simulink model "fuzzyLCSv1"  (R2021b)
settings: Solver=VariableStepAuto  StartTime=0.0  StopTime=10  RelTol=1e-3
undefined symbols (not defined in the file or in its folder): NewD, NewI, NewP
libraries: robotlib x3
settings Model: SimulationMode=accelerator  Creator=lucas  LastModifiedBy=lucas

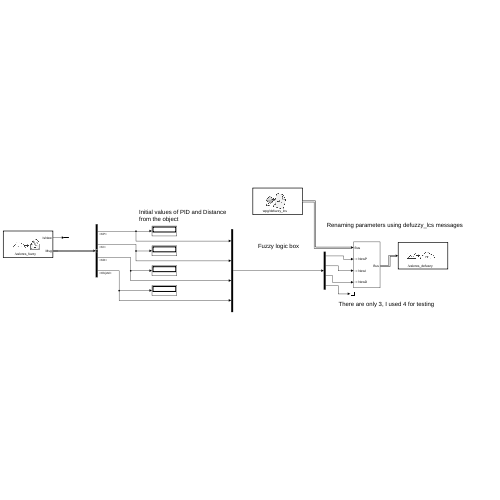
[thumbnail: Simulink's stored preview of the top-level diagram]
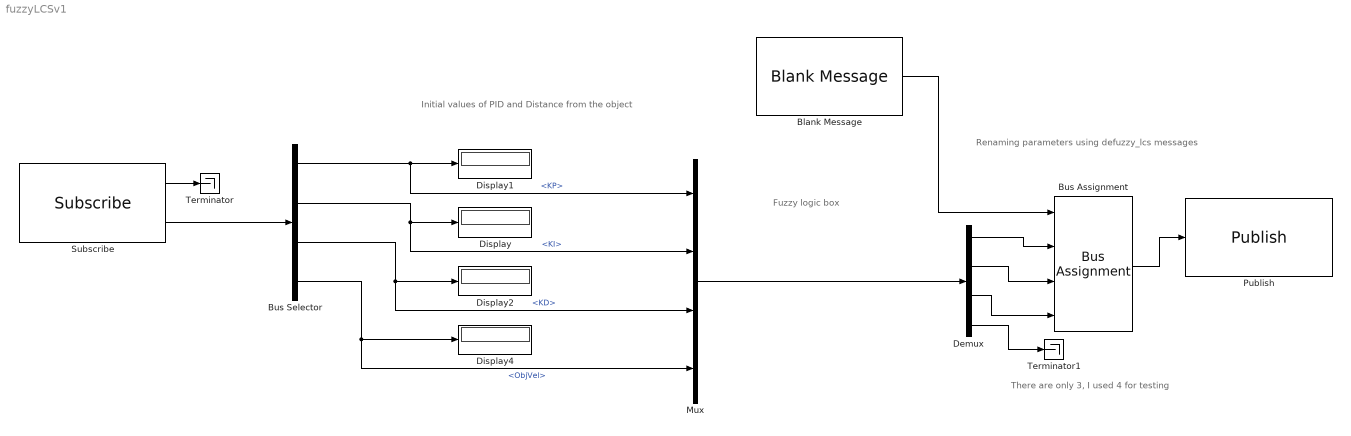
== system fuzzyLCSv1 ==
  note: Renaming parameters using defuzzy_lcs messages
  note: Initial values of PID and Distance
      | from the object
  note: Fuzzy logic box
  note: There are only 3, I used 4 for testing
  Blank Message : robotlib/Blank Message  messageClass=Message  entityType=wpg/defuzzy_lcs  messageType=wpg/defuzzy_lcs  SampleTime=inf  legacyBusStruct=off
  Bus Assignment : BusAssignment  AssignedSignals=NewP,NewI,NewD
  Bus Selector : BusSelector  OutputSignals=KP,KI,KD,ObjVel
  Demux : Demux
  Display{,1..2,4} (4 alike) : Display
      settings: Decimation=2
  Mux : Mux
  Publish : robotlib/Publish  topicSource=Specify your own  topic=/valores_defuzzy  messageType=wpg/defuzzy_lcs  legacyBusStruct=off  messageQueueLength=1
  Subscribe : robotlib/Subscribe  topicSource=Specify your own  topic=/valores_fuzzy  messageType=wpg/fuzzy_lcs  SampleTime=-1  legacyBusStruct=off  messageQueueLength=1
  Terminator : Terminator
  Terminator1 : Terminator
  wires:
  Subscribe/2 -> Bus Selector/1
  Subscribe/1 -> Terminator/1
  Bus Selector/1 -> Mux/1, Display1/1  "<KP>"
  Bus Selector/2 -> Mux/2, Display/1  "<KI>"
  Bus Selector/3 -> Mux/3, Display2/1  "<KD>"
  Blank Message/1 -> Bus Assignment/1
  Bus Assignment/1 -> Publish/1
  Bus Selector/4 -> Mux/4, Display4/1  "<ObjVel>"
  Mux/1 -> Demux/1
  Demux/1 -> Bus Assignment/2
  Demux/2 -> Bus Assignment/3
  Demux/3 -> Bus Assignment/4
  Demux/4 -> Terminator1/1
